simulink model "BidirectionalCurrentSystem"  (R2017a)
settings: Solver=ode45  StartTime=0.0  StopTime=10.0  RelTol=1e-3
undefined symbols (not defined in the file): Battery, Lib_PFSys_BiDirBattery_TMATS
libraries: Lib_PF_BusLoadDC_TMATS x4, Lib_PF_LineDC_TMATS x3, Lib_PF_BusSlackDC_TMATS x2, Lib_Solve_IterNRSolverJC_TMATS x1
settings Model: Creator=glthoma1  LastModifiedBy=glthoma1
settings DataIOCC: SaveFormat=StructureWithTime
settings OptimizationCC: LifeSpan=inf
settings DebuggingCC: SFExecutionAtInitializationDiag=none
settings HardwareCC: ProdBitPerSizeT=32  ProdBitPerPtrDiffT=32  ProdWordSize=32  ProdHWDeviceType=Specified
settings ConfigurationSet: Description=SimMechanics 2G

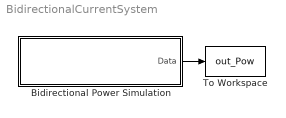
== system BidirectionalCurrentSystem ==
  Bidirectional Power Simulation : Subsystem
  To Workspace : ToWorkspace  VariableName=out_Pow  SaveFormat=Timeseries  SampleTime=-1
  wires:
  Bidirectional Power Simulation/1(Data) -> To Workspace/1

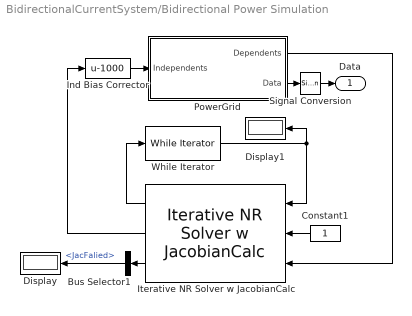
== system BidirectionalCurrentSystem/Bidirectional Power Simulation ==
  Bus Selector1 : BusSelector  OutputSignals=JacFalied
  Constant1 : Constant
  Display : Display
  Display1 : Display
  Ind Bias Corrector : Bias  Bias=-1000
  Iterative NR Solver w JacobianCalc : Lib_Solve_IterNRSolverJC_TMATS/Iterative NR Solver w JacobianCalc  SJac_Per_M=0.05*[1; -1]*[1 1]  SNR_IC_M=[10000 10000]+1000  SNR_DX_M=10  SNR_Mx_M=1e6  SNR_Mn_M=0.001  SJacobianAttempts_M=20  Cond_Limits_M=1e-4
  PowerGrid : Subsystem
  Signal Conversion : SignalConversion  OverrideOpt=off
  While Iterator : WhileIterator  MaxIters=100  WhileBlockType=do-while  ShowIterationPort=on
  Data : Outport
  wires:
  Ind Bias Corrector/1 -> PowerGrid/1(Independents)
  Bus Selector1/1 -> Display/1  "<JacFalied>"
  PowerGrid/1(Dependents) -> Iterative NR Solver w JacobianCalc/3
  While Iterator/1 -> Iterative NR Solver w JacobianCalc/1, Display1/1
  Iterative NR Solver w JacobianCalc/3 -> Bus Selector1/1
  Iterative NR Solver w JacobianCalc/1 -> While Iterator/1
  Constant1/1 -> Iterative NR Solver w JacobianCalc/2
  Iterative NR Solver w JacobianCalc/2 -> Ind Bias Corrector/1
  PowerGrid/2(Data) -> Signal Conversion/1
  Signal Conversion/1 -> Data/1

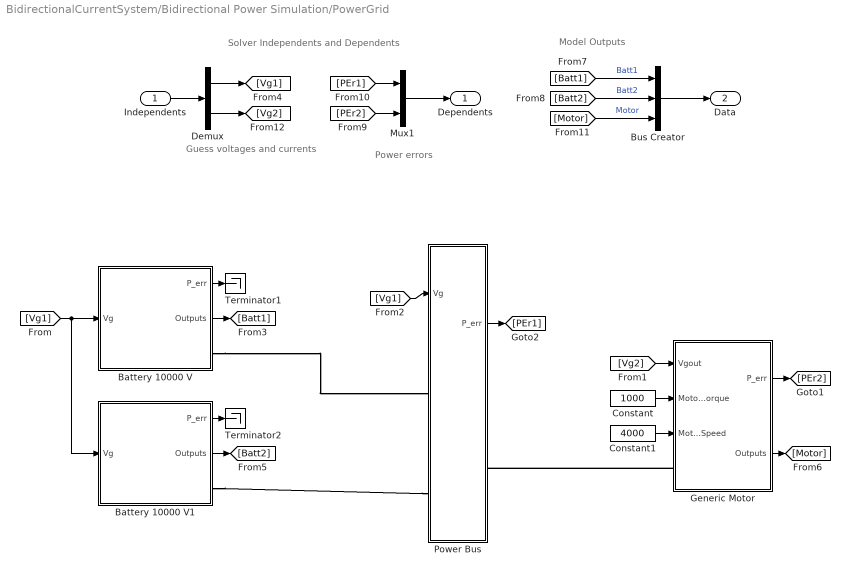
== system BidirectionalCurrentSystem/Bidirectional Power Simulation/PowerGrid ==
  note: Model Outputs
  note: Power errors
  note: Guess voltages
      | and currents
  note: Solver Independents and Dependents
  Independents : Inport
  Battery 10000 V : Subsystem  AncestorBlock=Lib_PFSys_BiDirBattery_TMATS/Battery  mask(Battery){Voltage_M=10000, Z_M=0.001}
      mask prompts: Voltage_M "Voltage_M - Nominal Voltage"; Z_M "Z_M - Impedance"
      mask help: This block takes in a nominal voltage input. It contains a slack bus and a battery impedance of 0.001 Ohms.
  Battery 10000 V1 : Subsystem  AncestorBlock=Lib_PFSys_BiDirBattery_TMATS/Battery  mask(Battery){Voltage_M=10100, Z_M=0.001}
      mask prompts: Voltage_M "Voltage_M - Nominal Voltage"; Z_M "Z_M - Impedance"
      mask help: This block takes in a nominal voltage input. It contains a slack bus and a battery impedance of 0.001 Ohms.
  Bus Creator : BusCreator  Inputs=3
  Constant : Constant  Value=1000
  Constant1 : Constant  Value=4000
  Demux : Demux  Outputs=2
  Generic Motor : Subsystem  AncestorBlock=Lib_PFSys_BiDirGenericMotor_TMATS/Generic Motor  mask(Motor){X_C_TorqueVec_M=[0 1000 10000], Y_C_SpeedVec_M=[0 500 5000], T_C_EffArray_M=[0.5 0.5 0.5; 0.5 1 1; 0.5 1 1], Z_M=0.01}
      mask prompts: X_C_TorqueVec_M "X_C_TorqueVec_M - Efficiency Table Torque Vector (X-axis)(nx1)"; Y_C_SpeedVec_M "Y_C_SpeedVec_M - Efficiency Table Speed Vector (Y-axis)(mx1)"; T_C_EffArray_M "T_C_EffArray_M - Efficiency Table Values (Eff = f(i, V)(nxm)"; Z_M "Z_M - Resistive Impedance"
      mask help: This block represents a generic motor with a standard resistive impedance of 0.01 Ohms and an efficiency table input.
  Mux1 : Mux  Inputs=2
  Power Bus : Subsystem  AncestorBlock=Lib_PFSys_BiDirBattery_TMATS/Battery  mask(Battery){Voltage_M=10000, Z_M=0.001}
      mask prompts: Voltage_M "Voltage_M - Nominal Voltage"; Z_M "Z_M - Impedance"
      mask help: This block takes in a nominal voltage input. It contains a slack bus and a battery impedance of 0.001 Ohms.
  Terminator1 : Terminator
  Terminator2 : Terminator
  Dependents : Outport
  Data : Outport  Port=2
  wires:
  Constant1/1 -> Generic Motor/3(MotorSpeed)
  [Vg2] -> Generic Motor/1(Vgout)
  Constant/1 -> Generic Motor/2(MotorTorque)
  Generic Motor/1(P_err) -> [PEr2]
  Battery 10000 V/1(P_err) -> Terminator1/1
  Demux/2 -> [Vg2]
  [PEr1] -> Mux1/1
  Mux1/1 -> Dependents/1
  Independents/1 -> Demux/1
  [PEr2] -> Mux1/2
  Demux/1 -> [Vg1]
  [Vg1] -> Battery 10000 V1/1(Vg), Battery 10000 V/1(Vg)
  Battery 10000 V1/1(P_err) -> Terminator2/1
  [Vg1] -> Power Bus/1(Vg)
  Battery 10000 V/2(Outputs) -> [Batt1]
  Battery 10000 V1/2(Outputs) -> [Batt2]
  Generic Motor/2(Outputs) -> [Motor]
  [Batt1] -> Bus Creator/1  "Batt1"
  [Batt2] -> Bus Creator/2  "Batt2"
  [Motor] -> Bus Creator/3  "Motor"
  Bus Creator/1 -> Data/1
  Power Bus/1(P_err) -> [PEr1]
  connections:
  Battery 10000 V/RConn1 -- Power Bus/LConn1
  Battery 10000 V1/RConn1 -- Power Bus/LConn2
  Generic Motor/LConn1 -- Power Bus/RConn1

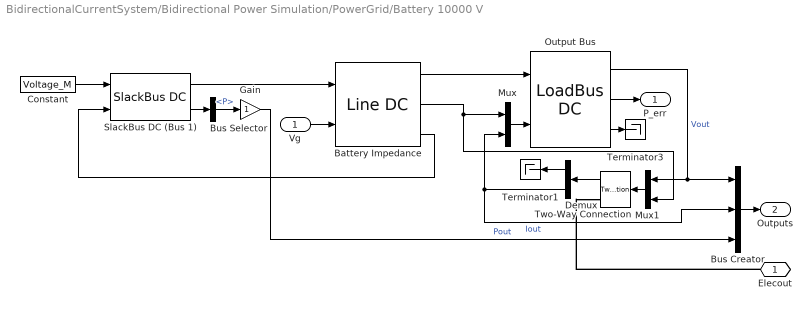
== system BidirectionalCurrentSystem/Bidirectional Power Simulation/PowerGrid/Battery 10000 V ==
  Vg : Inport
  Battery Impedance : Lib_PF_LineDC_TMATS/Line DC  R_M=Z_M
  Bus Creator : BusCreator  Inputs=3
  Bus Selector : BusSelector  OutputSignals=P
  Constant : Constant  Value=Voltage_M
  Demux : Demux  Outputs=2
  Gain : Gain
  Mux : Mux  Inputs=2
  Mux1 : Mux  Inputs=2
  Output Bus : Lib_PF_BusLoadDC_TMATS/LoadBus DC  PeInEN_M=off  P_M=0  BlkNm_M=double(gcb)
  SlackBus DC (Bus 1) : Lib_PF_BusSlackDC_TMATS/SlackBus DC
  Terminator1 : Terminator
  Terminator3 : Terminator
  Two-Way Connection : TwoWayConnection
  Elecout : PMIOPort  Port=1  Side=Right
  P_err : Outport
  Outputs : Outport  Port=2
  wires:
  Vg/1 -> Battery Impedance/2
  SlackBus DC (Bus 1)/1 -> Battery Impedance/1
  Battery Impedance/1 -> Output Bus/1
  Output Bus/1 -> Bus Creator/1, Mux1/1  "Vout"
  Output Bus/3 -> Terminator3/1
  SlackBus DC (Bus 1)/2 -> Bus Selector/1
  Constant/1 -> SlackBus DC (Bus 1)/1
  Output Bus/2 -> P_err/1
  Battery Impedance/3 -> SlackBus DC (Bus 1)/2
  Mux/1 -> Output Bus/2
  Demux/2 -> Bus Creator/2, Mux/2  "Iout"
  Bus Creator/1 -> Outputs/1
  Bus Selector/1 -> Gain/1  "<P>"
  Gain/1 -> Bus Creator/3  "Pout"
  Battery Impedance/2 -> Mux1/2, Mux/1
  Mux1/1 -> Two-Way Connection/1
  Two-Way Connection/1 -> Demux/1
  Demux/1 -> Terminator1/1
  connections:
  Elecout/RConn1 -- Two-Way Connection/RConn1

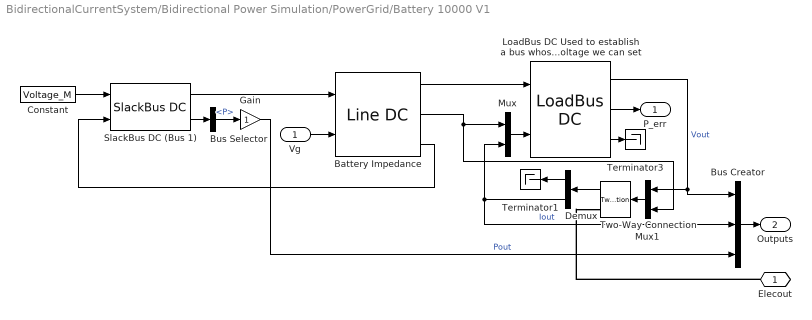
== system BidirectionalCurrentSystem/Bidirectional Power Simulation/PowerGrid/Battery 10000 V1 ==
  Vg : Inport
  Battery Impedance : Lib_PF_LineDC_TMATS/Line DC  R_M=Z_M
  Bus Creator : BusCreator  Inputs=3
  Bus Selector : BusSelector  OutputSignals=P
  Constant : Constant  Value=Voltage_M
  Demux : Demux  Outputs=2
  Gain : Gain
  LoadBus DC Used to establish a bus whose output voltage we can set : Lib_PF_BusLoadDC_TMATS/LoadBus DC  PeInEN_M=off  P_M=0  BlkNm_M=double(gcb)
  Mux : Mux  Inputs=2
  Mux1 : Mux  Inputs=2
  SlackBus DC (Bus 1) : Lib_PF_BusSlackDC_TMATS/SlackBus DC
  Terminator1 : Terminator
  Terminator3 : Terminator
  Two-Way Connection : TwoWayConnection
  Elecout : PMIOPort  Port=1  Side=Right
  P_err : Outport
  Outputs : Outport  Port=2
  wires:
  Vg/1 -> Battery Impedance/2
  SlackBus DC (Bus 1)/1 -> Battery Impedance/1
  Battery Impedance/1 -> LoadBus DC Used to establish a bus whose output voltage we can set/1
  LoadBus DC Used to establish a bus whose output voltage we can set/1 -> Bus Creator/1, Mux1/1  "Vout"
  LoadBus DC Used to establish a bus whose output voltage we can set/3 -> Terminator3/1
  SlackBus DC (Bus 1)/2 -> Bus Selector/1
  Constant/1 -> SlackBus DC (Bus 1)/1
  LoadBus DC Used to establish a bus whose output voltage we can set/2 -> P_err/1
  Battery Impedance/3 -> SlackBus DC (Bus 1)/2
  Mux/1 -> LoadBus DC Used to establish a bus whose output voltage we can set/2
  Demux/2 -> Bus Creator/2, Mux/2  "Iout"
  Bus Creator/1 -> Outputs/1
  Bus Selector/1 -> Gain/1  "<P>"
  Gain/1 -> Bus Creator/3  "Pout"
  Battery Impedance/2 -> Mux1/2, Mux/1
  Mux1/1 -> Two-Way Connection/1
  Two-Way Connection/1 -> Demux/1
  Demux/1 -> Terminator1/1
  connections:
  Elecout/RConn1 -- Two-Way Connection/RConn1

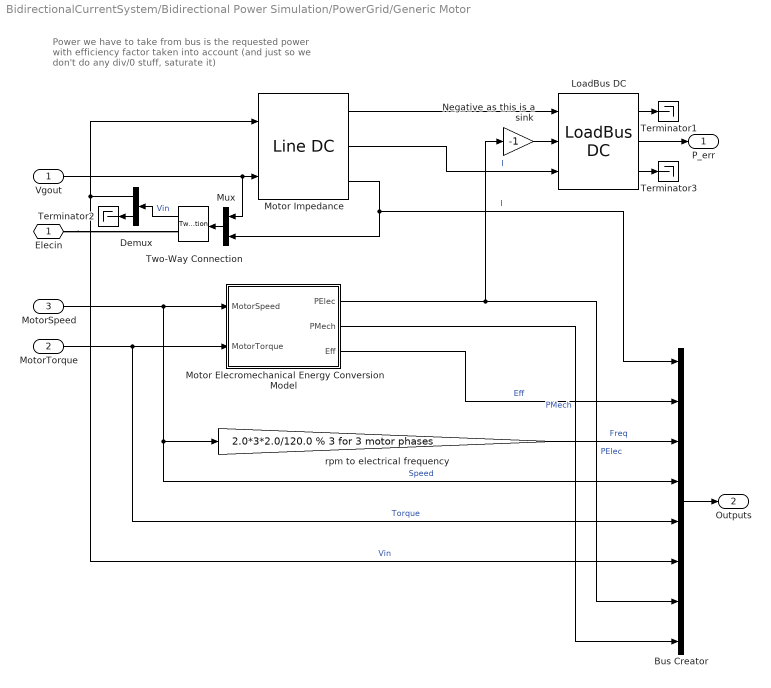
== system BidirectionalCurrentSystem/Bidirectional Power Simulation/PowerGrid/Generic Motor ==
  note: Power we have to take from bus is the requested power
      | with efficiency factor taken into account
      | (and just so we don't do any div/0 stuff, saturate it)
  Vgout : Inport
  MotorTorque : Inport  Port=2
  MotorSpeed : Inport  Port=3
  Bus Creator : BusCreator  Inputs=8
  Demux : Demux  Outputs=2
  LoadBus DC : Lib_PF_BusLoadDC_TMATS/LoadBus DC  PeInEN_M=on  P_M=-2  BlkNm_M=double(gcb)
  Motor Elecromechanical Energy Conversion Model : Subsystem
  Motor Impedance : Lib_PF_LineDC_TMATS/Line DC  R_M=Z_M
  Mux : Mux  Inputs=2
  Negative as this is a sink : Gain  Gain=-1
  Terminator1 : Terminator
  Terminator2 : Terminator
  Terminator3 : Terminator
  Two-Way Connection : TwoWayConnection
  rpm to electrical frequency : Gain  Gain=2.0*3*2.0/120.0 % 3 for 3 motor phases
  Elecin : PMIOPort  Port=1  Side=Left
  P_err : Outport
  Outputs : Outport  Port=2
  wires:
  Motor Elecromechanical Energy Conversion Model/2(PMech) -> Bus Creator/8  "PMech"
  Motor Elecromechanical Energy Conversion Model/3(Eff) -> Bus Creator/2  "Eff"
  Motor Elecromechanical Energy Conversion Model/1(PElec) -> Bus Creator/7, Negative as this is a sink/1  "PElec"
  LoadBus DC/1 -> Terminator1/1
  LoadBus DC/2 -> P_err/1
  Demux/1 -> Motor Impedance/1, Bus Creator/6  "Vin"
  LoadBus DC/3 -> Terminator3/1
  MotorSpeed/1 -> Motor Elecromechanical Energy Conversion Model/1(MotorSpeed), Bus Creator/4, rpm to electrical frequency/1  "Speed"
  MotorTorque/1 -> Motor Elecromechanical Energy Conversion Model/2(MotorTorque), Bus Creator/5  "Torque"
  rpm to electrical frequency/1 -> Bus Creator/3  "Freq"
  Bus Creator/1 -> Outputs/1
  Vgout/1 -> Mux/1, Motor Impedance/2
  Motor Impedance/1 -> LoadBus DC/1
  Motor Impedance/3 -> Mux/2, Bus Creator/1  "I"
  Motor Impedance/2 -> LoadBus DC/3  "I"
  Negative as this is a sink/1 -> LoadBus DC/2
  Two-Way Connection/1 -> Demux/1  "Vin"
  Demux/2 -> Terminator2/1
  Mux/1 -> Two-Way Connection/1
  connections:
  Elecin/RConn1 -- Two-Way Connection/RConn1

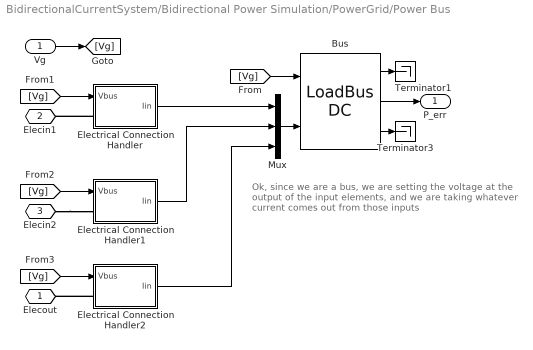
== system BidirectionalCurrentSystem/Bidirectional Power Simulation/PowerGrid/Power Bus ==
  note: Ok, since we are a bus, we are setting the voltage at the
      | output of the input elements, and we are taking whatever
      | current comes out from those inputs
  Vg : Inport
  Bus : Lib_PF_BusLoadDC_TMATS/LoadBus DC  PeInEN_M=off  P_M=0  BlkNm_M=double(gcb)
  Electrical Connection Handler : Subsystem
  Electrical Connection Handler1 : Subsystem
  Electrical Connection Handler2 : Subsystem
  Mux : Mux  Inputs=3
  Terminator1 : Terminator
  Terminator3 : Terminator
  Elecout : PMIOPort  Port=1  Side=Right
  Elecin1 : PMIOPort  Port=2  Side=Left
  Elecin2 : PMIOPort  Port=3  Side=Left
  P_err : Outport
  wires:
  Bus/3 -> Terminator3/1
  Bus/2 -> P_err/1
  Mux/1 -> Bus/2
  [Vg] -> Bus/1
  Vg/1 -> [Vg]
  Bus/1 -> Terminator1/1
  [Vg] -> Electrical Connection Handler/1(Vbus)
  Electrical Connection Handler/1(Iin) -> Mux/1
  [Vg] -> Electrical Connection Handler1/1(Vbus)
  Electrical Connection Handler1/1(Iin) -> Mux/2
  [Vg] -> Electrical Connection Handler2/1(Vbus)
  Electrical Connection Handler2/1(Iin) -> Mux/3
  connections:
  Electrical Connection Handler/LConn1 -- Elecin1/RConn1
  Elecin2/RConn1 -- Electrical Connection Handler1/LConn1
  Electrical Connection Handler2/LConn1 -- Elecout/RConn1

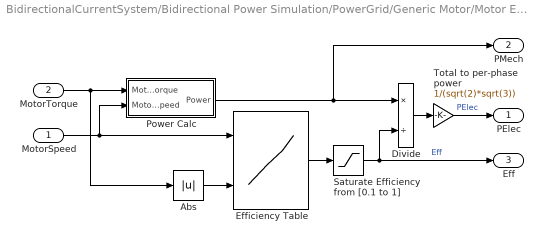
== system BidirectionalCurrentSystem/Bidirectional Power Simulation/PowerGrid/Generic Motor/Motor Elecromechanical Energy Conversion Model ==
  MotorSpeed : Inport
  MotorTorque : Inport  Port=2
  Abs : Abs
  Divide : Product  Inputs=*/
  Efficiency Table : Lookup_n-D  BreakpointsForDimension1=X_C_TorqueVec_M  BreakpointsForDimension2=Y_C_SpeedVec_M  Table=T_C_EffArray_M  ExtrapMethod=Clip  InternalRulePriority=Speed  RndMeth=Simplest  InputSameDT=on
  Power Calc : Subsystem
  Saturate Efficiency from [0.1 to 1] : Saturate  UpperLimit=1  LowerLimit=0.1
  Total to per-phase power : Gain  Gain=1/(sqrt(2)*sqrt(3))
  PElec : Outport
  PMech : Outport  Port=2
  Eff : Outport  Port=3
  wires:
  MotorSpeed/1 -> Efficiency Table/1, Power Calc/2(MotorSpeed)
  MotorTorque/1 -> Power Calc/1(MotorTorque), Abs/1
  Power Calc/1(Power) -> Divide/1, PMech/1
  Divide/1 -> Total to per-phase power/1
  Total to per-phase power/1 -> PElec/1  "PElec"
  Abs/1 -> Efficiency Table/2
  Saturate Efficiency from [0.1 to 1]/1 -> Divide/2, Eff/1  "Eff"
  Efficiency Table/1 -> Saturate Efficiency from [0.1 to 1]/1

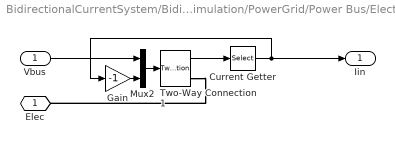
== system BidirectionalCurrentSystem/Bidirectional Power Simulation/PowerGrid/Power Bus/Electrical Connection Handler ==
  Vbus : Inport
  Current Getter : Selector  IndexOptions=Index vector (dialog)  Indices=2  OutputSizes=1
  Gain : Gain  Gain=-1
  Mux2 : Mux  Inputs=2
  Two-Way Connection1 : TwoWayConnection
  Elec : PMIOPort  Port=1  Side=Left
  Iin : Outport
  wires:
  Gain/1 -> Mux2/2
  Mux2/1 -> Two-Way Connection1/1
  Two-Way Connection1/1 -> Current Getter/1
  Current Getter/1 -> Iin/1, Gain/1
  Vbus/1 -> Mux2/1
  connections:
  Two-Way Connection1/RConn1 -- Elec/RConn1

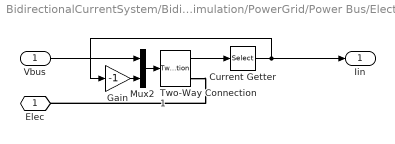
== system BidirectionalCurrentSystem/Bidirectional Power Simulation/PowerGrid/Power Bus/Electrical Connection Handler1 ==
  Vbus : Inport
  Current Getter : Selector  IndexOptions=Index vector (dialog)  Indices=2  OutputSizes=1
  Gain : Gain  Gain=-1
  Mux2 : Mux  Inputs=2
  Two-Way Connection1 : TwoWayConnection
  Elec : PMIOPort  Port=1  Side=Left
  Iin : Outport
  wires:
  Gain/1 -> Mux2/2
  Mux2/1 -> Two-Way Connection1/1
  Two-Way Connection1/1 -> Current Getter/1
  Current Getter/1 -> Iin/1, Gain/1
  Vbus/1 -> Mux2/1
  connections:
  Two-Way Connection1/RConn1 -- Elec/RConn1

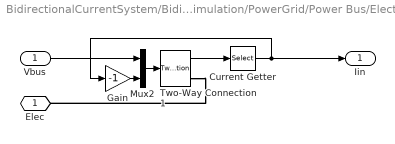
== system BidirectionalCurrentSystem/Bidirectional Power Simulation/PowerGrid/Power Bus/Electrical Connection Handler2 ==
  Vbus : Inport
  Current Getter : Selector  IndexOptions=Index vector (dialog)  Indices=2  OutputSizes=1
  Gain : Gain  Gain=-1
  Mux2 : Mux  Inputs=2
  Two-Way Connection1 : TwoWayConnection
  Elec : PMIOPort  Port=1  Side=Left
  Iin : Outport
  wires:
  Gain/1 -> Mux2/2
  Mux2/1 -> Two-Way Connection1/1
  Two-Way Connection1/1 -> Current Getter/1
  Current Getter/1 -> Iin/1, Gain/1
  Vbus/1 -> Mux2/1
  connections:
  Two-Way Connection1/RConn1 -- Elec/RConn1

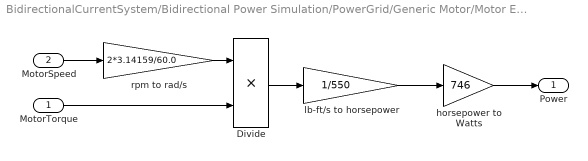
== system BidirectionalCurrentSystem/Bidirectional Power Simulation/PowerGrid/Generic Motor/Motor Elecromechanical Energy Conversion Model/Power Calc ==
  MotorTorque : Inport
  MotorSpeed : Inport  Port=2
  Divide : Product  Inputs=**
  horsepower to Watts : Gain  Gain=746
  lb-ft/s to horsepower : Gain  Gain=1/550
  rpm to rad/s : Gain  Gain=2*3.14159/60.0
  Power : Outport
  wires:
  horsepower to Watts/1 -> Power/1
  rpm to rad/s/1 -> Divide/1
  MotorTorque/1 -> Divide/2
  lb-ft/s to horsepower/1 -> horsepower to Watts/1
  Divide/1 -> lb-ft/s to horsepower/1
  MotorSpeed/1 -> rpm to rad/s/1
